simulink model "flightController"  (R2019b)
settings: Solver=ode3  StartTime=0  StopTime=TFinal  FixedStep=Ts  RelTol=1e-3  EnableMultiTasking=on
values from neighbouring files (symbols this model uses):
  A = dsys.A    [LQRCtrl.m]
  B = dsys.B    [LQRCtrl.m]
  Bd = A(1:12,13:18)    [LQRCtrl.m]
  C = dsys.C    [LQRCtrl.m]
  K = dlqr(Alqr, Blqr, Qlqr, R)    [LQRCtrl.m]
  M = pinv(M)    [LQRCtrl.m]
  Ro = eye(6)    [LQRCtrl.m]
undefined symbols (not defined in the file or in its folder): Controller, Discrete, g, Time, Ts, Vehicle
libraries: ctrlSharedLib x1
settings Model: ExtModeTrigDuration=80  Creator=The MathWorks, Inc.  LastModifiedBy=DKKim
settings SolverCC: MinimalZcImpactIntegration=on
settings DataIOCC: LimitDataPoints=on  SaveFormat=Array  ReturnWorkspaceOutputs=off
settings OptimizationCC: BlockReduction=off  EnhancedBackFolding=on  PassReuseOutputArgsAs=Individual arguments  ZeroExternalMemoryAtStartup=off  ZeroInternalMemoryAtStartup=off  MaxStackSize=64  OptimizeBlockOrder=speed  DifferentSizesBufferReuse=on  OptimizationCustomize=off  EfficientTunableParamExpr=on
settings DebuggingCC: AlgebraicLoopMsg=none  ParameterPrecisionLossMsg=none  ParameterTunabilityLossMsg=error  UnconnectedInputMsg=none  UnconnectedOutputMsg=none  UnconnectedLineMsg=none  BusObjectLabelMismatch=error  SFUnexpectedBacktrackingDiag=warning  SFNoUnconditionalDefaultTransitionDiag=warning  SFExecutionAtInitializationDiag=none  ArithmeticOperatorsInVariantConditions=warning
settings HardwareCC: ProdBitPerPointer=32  ProdBitPerSizeT=32  ProdBitPerPtrDiffT=32  ProdLargestAtomicInteger=Long  ProdWordSize=32  ProdHWDeviceType=ARM Compatible->ARM 9
settings ModelReferenceCC: ModelReferenceNumInstancesAllowed=Single  PropagateSignalLabelsOutOfModel=off
settings SFSimCC: SimUseLocalCustomCode=off  MATLABDynamicMemAlloc=off  CustomCodeUndefinedFunction=UseInterfaceOnly
settings RTWCC: SystemTargetFile=ert.tlc  HardwareBoard=PARROT Mambo  TLCOptions=-aInlineSetEventsForThisBaseRateFcn=TLC_FALSE -aSuppressMultiTaskScheduler=TLC_FALSE -aRateBasedStepFcn=1  TemplateMakefile=ert_default_tmf  GenerateReport=on  RTWUseLocalCustomCode=off  Toolchain=Sourcery G++ Lite GNU Toolchain for Drones  IncludeHyperlinkInReport=on  LaunchReport=on  GenerateTraceInfo=on  GenerateTraceReport=on  GenerateTraceReportSl=on  GenerateTraceReportSf=on  GenerateTraceReportEml=on
settings CodeAppCC: ForceParamTrailComments=on  IgnoreCustomStorageClasses=off  MaxIdLength=63  OperatorAnnotations=on  SimulinkDataObjDesc=on  SFDataObjDesc=on  InsertBlockDesc=on
settings ERTTargetCC: MatFileLogging=on
settings ConfigComp: CovMetricSettings=dw  CovHtmlReporting=on  CovSaveCumulativeToWorkspaceVar=on  CovSaveSingleToWorkspaceVar=on  CovExternalEMLEnable=off  CovSFcnEnable=off

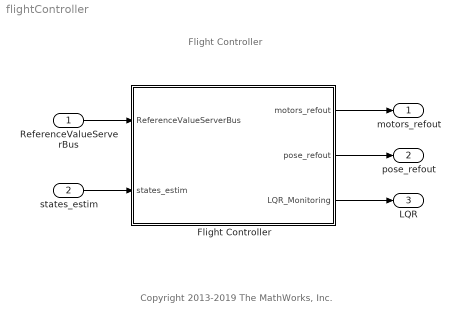
== system flightController ==
  note: Flight Controller
  note: Copyright 2013-2019 The MathWorks, Inc.
  ReferenceValueServerBus : Inport  OutDataTypeStr=Bus: CommandBus  BusOutputAsStruct=on
  states_estim : Inport  Port=2  OutDataTypeStr=Bus: statesEstim_t  BusOutputAsStruct=on
  Flight Controller : Subsystem
  motors_refout : Outport  VectorParamsAs1DForOutWhenUnconnected=off
  pose_refout : Outport  Port=2  VectorParamsAs1DForOutWhenUnconnected=off
  LQR : Outport  Port=3
  wires:
  ReferenceValueServerBus/1 -> Flight Controller/1(ReferenceValueServerBus)
  states_estim/1 -> Flight Controller/2(states_estim)
  Flight Controller/2(pose_refout) -> pose_refout/1
  Flight Controller/1(motors_refout) -> motors_refout/1
  Flight Controller/3(LQR_Monitoring) -> LQR/1

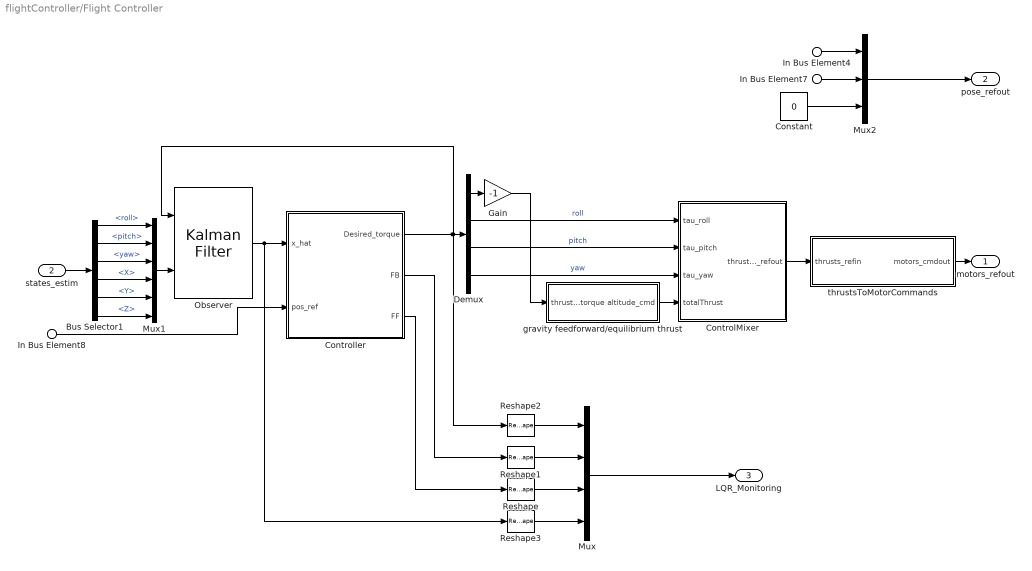
== system flightController/Flight Controller ==
  In Bus Element4 : Inport  PortName=ReferenceValueServerBus  Element=pos_ref
  In Bus Element8 : Inport  PortName=ReferenceValueServerBus  Element=pos_ref
  In Bus Element7 : Inport  PortName=ReferenceValueServerBus  Element=orient_ref
  states_estim : Inport  Port=2
  Bus Selector1 : BusSelector  OutputSignals=roll,pitch,yaw,X,Y,Z
  Constant : Constant  Value=0  OutDataTypeStr=single
  ControlMixer : Subsystem
  Controller : Subsystem
  Demux : Demux
  Gain : Gain  Gain=-1
  Mux : Mux
  Mux1 : Mux  Inputs=6
  Mux2 : Mux  Inputs=3
  Observer : ctrlSharedLib/Kalman Filter  TimeDomain=Discrete-Time  UseCurrentEstimator=on  ModelSource=Individual A, B, C, D matrices  ModelSourceVariable=ss(0.95,1,1,0,1)  A=A  B=B  C=C  D=0  NumberOfStates=1  NumberOfInputs=1  NumberOfOutputs=1  InitialEstimateSource=Dialog  X0=0  P0=10  UseK=off  UseGH=off  NumberOfProcessNoiseInputs=1  G=1  TimeInvariantG=on  H=0  TimeInvariantH=on  Q=Q  TimeInvariantQ=on  R=Ro  TimeInvariantR=on  N=0  TimeInvariantN=on  AddInputPort=on  AddEnablePort=off  OutputEstimatedY=off  OutputP=off  Ts=Ts
      settings: SourceProductBaseCode=CT
  Reshape{,1..3} (4 alike) : Reshape
  gravity feedforward/equilibrium thrust : Subsystem
  thrustsToMotorCommands : Subsystem
  motors_refout : Outport  VectorParamsAs1DForOutWhenUnconnected=off
  pose_refout : Outport  Port=2  VectorParamsAs1DForOutWhenUnconnected=off
  LQR_Monitoring : Outport  Port=3
  wires:
  thrustsToMotorCommands/1(motors_cmdout) -> motors_refout/1
  ControlMixer/1(thrusts_refout) -> thrustsToMotorCommands/1(thrusts_refin)
  gravity feedforward/equilibrium thrust/1(altitude_cmd) -> ControlMixer/4(totalThrust)
  Mux2/1 -> pose_refout/1
  In Bus Element4/1 -> Mux2/1
  In Bus Element7/1 -> Mux2/2
  Demux/3 -> ControlMixer/2(tau_pitch)  "pitch"
  Gain/1 -> gravity feedforward/equilibrium thrust/1(thrust_torque)
  Demux/4 -> ControlMixer/3(tau_yaw)  "yaw"
  Demux/2 -> ControlMixer/1(tau_roll)  "roll"
  states_estim/1 -> Bus Selector1/1
  Bus Selector1/3 -> Mux1/3  "<yaw>"
  Bus Selector1/4 -> Mux1/4  "<X>"
  Bus Selector1/5 -> Mux1/5  "<Y>"
  Bus Selector1/6 -> Mux1/6  "<Z>"
  Mux1/1 -> Observer/2
  Demux/1 -> Gain/1
  Constant/1 -> Mux2/3
  Controller/1(Desired_torque) -> Observer/1, Reshape2/1, Demux/1
  Observer/1 -> Reshape3/1, Controller/1(x_hat)
  Bus Selector1/2 -> Mux1/2  "<pitch>"
  Bus Selector1/1 -> Mux1/1  "<roll>"
  Mux/1 -> LQR_Monitoring/1
  In Bus Element8/1 -> Controller/2(pos_ref)
  Controller/3(FF) -> Reshape/1
  Controller/2(FB) -> Reshape1/1
  Reshape/1 -> Mux/3
  Reshape1/1 -> Mux/2
  Reshape2/1 -> Mux/1
  Reshape3/1 -> Mux/4

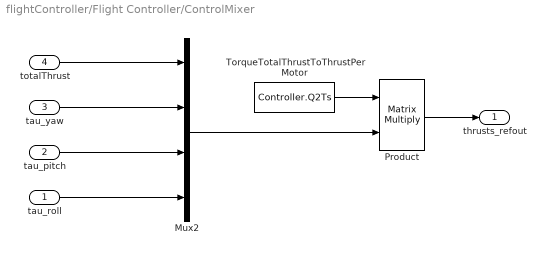
== system flightController/Flight Controller/ControlMixer ==
  tau_roll : Inport
  tau_pitch : Inport  Port=2
  tau_yaw : Inport  Port=3
  totalThrust : Inport  Port=4
  Mux2 : Mux
  Product : Product  Multiplication=Matrix(*)  RndMeth=Zero
  TorqueTotalThrustToThrustPerMotor : Constant  Value=Controller.Q2Ts  OutDataTypeStr=single
  thrusts_refout : Outport  VectorParamsAs1DForOutWhenUnconnected=off
  wires:
  Product/1 -> thrusts_refout/1
  totalThrust/1 -> Mux2/1
  TorqueTotalThrustToThrustPerMotor/1 -> Product/1
  Mux2/1 -> Product/2
  tau_yaw/1 -> Mux2/2
  tau_pitch/1 -> Mux2/3
  tau_roll/1 -> Mux2/4

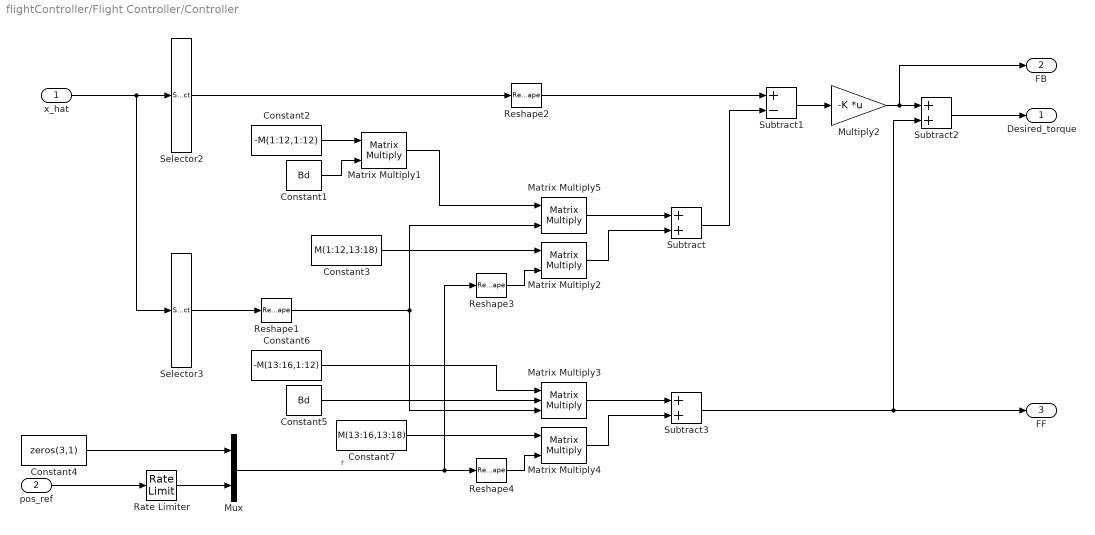
== system flightController/Flight Controller/Controller ==
  x_hat : Inport
  pos_ref : Inport  Port=2
  Constant1 : Constant  Value=Bd  OutDataTypeStr=single
  Constant2 : Constant  Value=-M(1:12,1:12)  OutDataTypeStr=single
  Constant3 : Constant  Value=M(1:12,13:18)  OutDataTypeStr=single
  Constant4 : Constant  Value=zeros(3,1)  OutDataTypeStr=single
  Constant5 : Constant  Value=Bd  OutDataTypeStr=single
  Constant6 : Constant  Value=-M(13:16,1:12)  OutDataTypeStr=single
  Constant7 : Constant  Value=M(13:16,13:18)  OutDataTypeStr=single
  Matrix Multiply{1..2,4..5} (4 alike) : Product  Multiplication=Matrix(*)
  Matrix Multiply3 : Product  Inputs=3  Multiplication=Matrix(*)
  Multiply2 : Gain  Gain=-K  Multiplication=Matrix(K*u)
  Mux : Mux  Inputs=2
  Rate Limiter : RateLimiter  RisingSlewLimit=2  FallingSlewLimit=-2  SampleTimeMode=inherited
  Reshape{1..4} (4 alike) : Reshape  OutputDimensionality=Column vector (2-D)
  Selector2 : Selector  InputPortWidth=18  IndexOptions=Index vector (dialog)  Indices=[1:12]  OutputSizes=1
  Selector3 : Selector  InputPortWidth=18  IndexOptions=Index vector (dialog)  Indices=[13:18]  OutputSizes=1
  Subtract : Sum
  Subtract1 : Sum  Inputs=+-
  Subtract2 : Sum
  Subtract3 : Sum
  Desired_torque : Outport
  FB : Outport  Port=2
  FF : Outport  Port=3
  wires:
  Subtract1/1 -> Multiply2/1
  Selector2/1 -> Reshape2/1
  Selector3/1 -> Reshape1/1
  Constant2/1 -> Matrix Multiply1/1
  Constant1/1 -> Matrix Multiply1/2
  Reshape1/1 -> Matrix Multiply5/2, Matrix Multiply3/3
  Matrix Multiply2/1 -> Subtract/2
  Constant3/1 -> Matrix Multiply2/1
  Reshape2/1 -> Subtract1/1
  Subtract/1 -> Subtract1/2
  Multiply2/1 -> FB/1, Subtract2/1
  Subtract2/1 -> Desired_torque/1
  x_hat/1 -> Selector3/1, Selector2/1
  Constant6/1 -> Matrix Multiply3/1
  Subtract3/1 -> FF/1, Subtract2/2
  Constant7/1 -> Matrix Multiply4/1
  Matrix Multiply3/1 -> Subtract3/1
  Matrix Multiply4/1 -> Subtract3/2
  Constant5/1 -> Matrix Multiply3/2
  Matrix Multiply1/1 -> Matrix Multiply5/1
  Matrix Multiply5/1 -> Subtract/1
  Mux/1 -> Reshape3/1, Reshape4/1  "r"
  Reshape3/1 -> Matrix Multiply2/2
  Reshape4/1 -> Matrix Multiply4/2
  Constant4/1 -> Mux/1
  pos_ref/1 -> Rate Limiter/1
  Rate Limiter/1 -> Mux/2

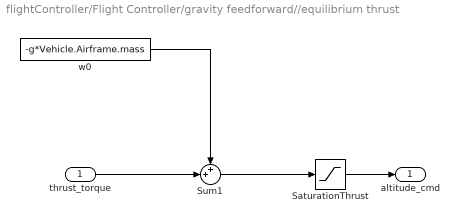
== system flightController/Flight Controller/gravity feedforward//equilibrium thrust ==
  thrust_torque : Inport
  SaturationThrust : Saturate  UpperLimit=4*Controller.totalThrustMaxRelative*Controller.motorsThrustPerMotorMax  LowerLimit=-4*Controller.totalThrustMaxRelative*Controller.motorsThrustPerMotorMax  OutDataTypeStr=single
  Sum1 : Sum  Inputs=++|  AccumDataTypeStr=single  OutDataTypeStr=single  SaturateOnIntegerOverflow=on
  w0 : Constant  Value=-g*Vehicle.Airframe.mass  OutDataTypeStr=single  SampleTime=Ts
  altitude_cmd : Outport  VectorParamsAs1DForOutWhenUnconnected=off
  wires:
  w0/1 -> Sum1/1
  SaturationThrust/1 -> altitude_cmd/1
  Sum1/1 -> SaturationThrust/1
  thrust_torque/1 -> Sum1/2

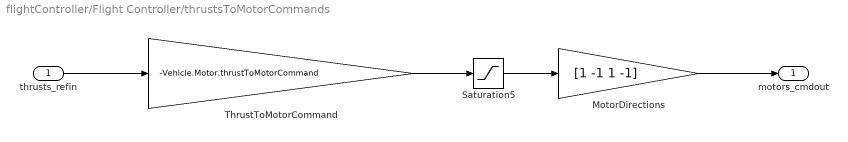
== system flightController/Flight Controller/thrustsToMotorCommands ==
  thrusts_refin : Inport
  MotorDirections : Gain  Gain=[1 -1 1 -1]
  Saturation5 : Saturate  UpperLimit=Vehicle.Motor.maxLimit  LowerLimit=Vehicle.Motor.minLimit
  ThrustToMotorCommand : Gain  Gain=-Vehicle.Motor.thrustToMotorCommand
  motors_cmdout : Outport  VectorParamsAs1DForOutWhenUnconnected=off
  wires:
  Saturation5/1 -> MotorDirections/1
  MotorDirections/1 -> motors_cmdout/1
  ThrustToMotorCommand/1 -> Saturation5/1
  thrusts_refin/1 -> ThrustToMotorCommand/1
